simulink model "Commander_Stabilizer_QBot2e_Leader"  (Simulink 10.1)
settings: Solver=ode2  StartTime=0.0  StopTime=inf  FixedStep=0.002  RelTol=1e-3  EnableMultiTasking=on
model workspace (MAT data in the model file):
  Sig = Simulink.Signal
  Sig.DataType = 'auto'
  Sig.Dimensions = -1
  Sig.DimensionsMode = 'auto'
  Sig.Complexity = 'auto'
  Sig.SampleTime = -1
  Sig.SamplingMode = 'auto'
  video_step_size = 0.06
undefined symbols (not defined in the file): datetime, HIL, m, QBot2e_Commander_, QBot2e_Stabilizer_, saved_data
libraries: quarc_library x25, simulink x7
settings Model: Creator=Admin  LastModifiedBy=glai  SimulationMode=external
settings SolverCC: PositivePriorityOrder=on
settings DataIOCC: SaveFormat=Dataset
settings OptimizationCC: LifeSpan=auto
settings DebuggingCC: UnderspecifiedInitializationDetection=Simplified  MergeDetectMultiDrivingBlocksExec=error  ParameterPrecisionLossMsg=none
settings HardwareCC: ProdLargestAtomicInteger=Long  ProdLargestAtomicFloat=Double  ProdIntDivRoundTo=Zero  ProdEndianess=LittleEndian  ProdHWDeviceType=ARM Compatible->ARM Cortex
settings ModelReferenceCC: PropagateSignalLabelsOutOfModel=on
settings RTWCC: Description=QUARC Linux Raspberry Pi 3 Target (QBot 2e) Using Toolchain  SystemTargetFile=quarc_linux_pi_3.tlc  TemplateMakefile=quarc_default_tmf  Toolchain=QUARC linux_pi_3 | gmake (64-bit Windows)  BuildConfiguration=Faster Runs
settings STFCustomTargetCC: ConcurrentExecutionCompliant=on  UseToolchainInfoCompliant=on  SystemTargetFile=quarc_linux_pi_3.tlc
settings GRTTargetCC: ParMdlRefBuildCompliant=off  CompOptLevelCompliant=off  MatFileLogging=off  CPPClassGenCompliant=off  ExtMode=on  ExtModeMexFile=quarc_comm  ExtModeMexArgs='-w -d /tmp -uri %u -URI_Leader tcpip://localhost:18002 -URI_Host tcpip://192.168.2.H:18001','tcpip://192.168.2.Y:17001'
settings ConfigComp: CovHtmlReporting=off

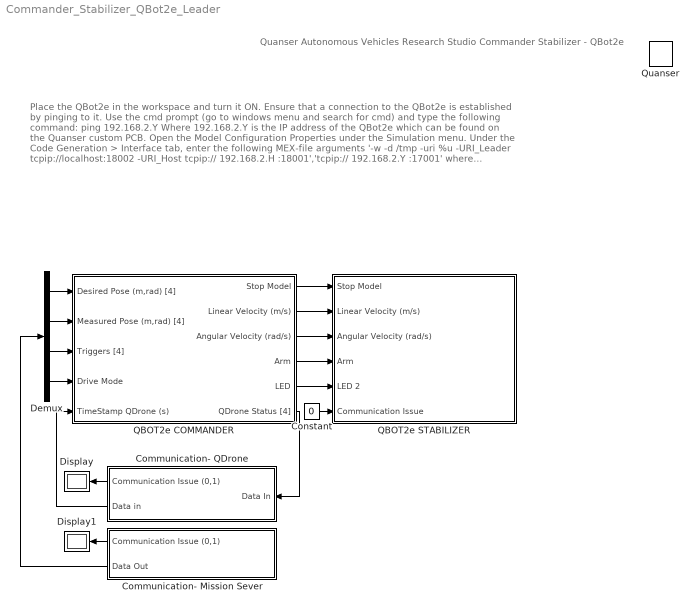
== system Commander_Stabilizer_QBot2e_Leader ==
  note: Quanser Autonomous Vehicles Research Studio
      | Commander Stabilizer - QBot2e
  note: Place the QBot2e in the workspace and turn it ON.
      | Ensure that a connection to the QBot2e is established by pinging to it. Use the cmd prompt (go to windows menu and search for cmd) and type the following command:
      | ping 192.168.2.Y
      | Where 192.168.2.Y is the IP address of the QBot2e which can be found on the Quanser custom PCB.
      |
      | Open the Model Configuration Properties under the Simulation menu.
      |
      | Under the Code Generation > Interface tab, enter the following MEX-file arguments
      | '-w -d /tmp -uri %u -URI_Leader tcpip://localhost:18002 -URI_Host tcpip:// 192.168.2.H :18001','tcpip:// 192.168.2.Y :17001'
      | where 192.168.2.H is the IP address of the ground control station PC (should be 192.168.2.5 by default), 192.168.2.Y is the IP address of the QBot2e which can be found on the custom Quanser PCB.
      |
      | Under the QUARC menu, click on Build .
      | NOTE : Ensure that the corresponding Mission_Server_Leader_Follower is running first before continuing.
      |
      | Under the QUARC menu, click on Start .
      |
      | You will hear a sequence of beeps, which indicate that the model has started running on the QBot 2e.
  "Communication- Mission Sever " : Subsystem
  Communication- QDrone : Subsystem
  Constant : Constant  Value=0
  Demux : Demux  Outputs=[ 4 4 4 1]
  Display : Display
  Display1 : Display
  QBOT2e COMMANDER : Subsystem
  QBOT2e STABILIZER : Subsystem
  Quanser : quarc_library/Logos/Quanser
  wires:
  QBOT2e COMMANDER/1(Stop Model) -> QBOT2e STABILIZER/1(Stop Model)
  QBOT2e COMMANDER/3(Angular Velocity (rad/s)) -> QBOT2e STABILIZER/3(Angular Velocity (rad/s))
  QBOT2e COMMANDER/4(Arm) -> QBOT2e STABILIZER/4(Arm)
  QBOT2e COMMANDER/2(Linear Velocity (m/s)) -> QBOT2e STABILIZER/2(Linear Velocity (m/s))
  QBOT2e COMMANDER/5(LED) -> QBOT2e STABILIZER/5(LED 2)
  "Communication- Mission Sever "/2(Data Out) -> Demux/1
  Demux/2 -> QBOT2e COMMANDER/2(Measured Pose (m,rad) [4])
  Demux/1 -> QBOT2e COMMANDER/1(Desired Pose (m,rad) [4])
  Constant/1 -> QBOT2e STABILIZER/6(Communication Issue)
  Demux/3 -> QBOT2e COMMANDER/3(Triggers [4])
  Demux/4 -> QBOT2e COMMANDER/4("Drive Mode ")
  QBOT2e COMMANDER/6(QDrone Status [4]) -> Communication- QDrone/1(Data In)
  Communication- QDrone/1(Communication Issue (0,1)) -> Display/1
  "Communication- Mission Sever "/1(Communication Issue (0,1)) -> Display1/1
  Communication- QDrone/2(Data in) -> QBOT2e COMMANDER/5(TimeStamp QDrone (s))

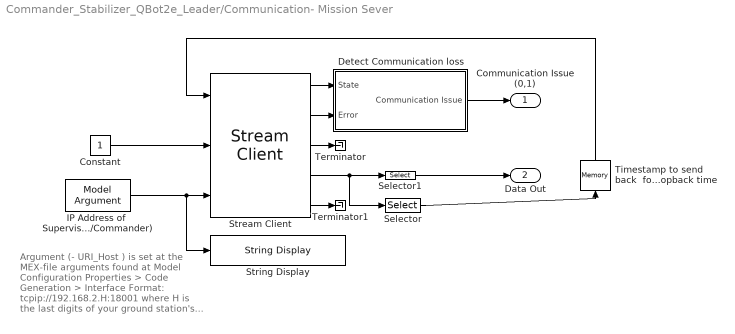
== system Commander_Stabilizer_QBot2e_Leader/Communication- Mission Sever  ==
  note: Argument (- URI_Host ) is set at the MEX-file arguments found at Model Configuration Properties > Code Generation > Interface
      |
      | Format:
      | tcpip://192.168.2.H:18001
      | where H is the last digits of your ground station's IP address (use ipconfig in a command prompt to find it out).
  Constant : Constant
  Detect Communication loss : Subsystem
  IP Address of  Supervisory Model (Mission Operator/Commander) : quarc_library/Sources/Signals/Model Argument  argument_name=URI_Host  has_value=on  data_type_mode=Specify via dialog  data_type=char  max_length=80  default_value=0  default_string=tcpip://192.168.2.H:18001  variable_size=off
      settings: AttributesFormatString=(-%<argument_name>)  SourceProductName=QUARC Targets
  Selector : Selector  InputPortWidth=14  IndexOptions=Index vector (dialog)  Indices=[14]  OutputSizes=1
  Selector1 : Selector  InputPortWidth=14  IndexOptions=Index vector (dialog)  Indices=[1:13]  OutputSizes=1
  Stream Client : quarc_library/Communications/Basic/Stream Client  uri_source=External input port  uri=tcpip://localhost:18999  apply_uri_to_all_configs=on  send_buffer_size=1460  receive_buffer_size=1460  byte_order=little endian (Intel - LSB first)  optimization=Minimum latency  send_options=Send most recent data  receive_options=Receive most recent data  default_value=zeros(1,14)  sample_time=qc_get_step_size  active=off  implementation=Use blocking I/O in a separate thread  send_fifo_size=1  receive_fifo_size=1  send_priority=0  receive_priority=0  send_dimensions=off  receive_dimensions=off  max_dimensions=-1  data_type=double  type_expr=BusObject
      settings: SourceProductName=The database C:\Users\user\AppData\Roaming\MathWorks\MATLAB\R2017a\slblocks_master.db is locked, or a table in the database is locked. (database is locked)
  String Display : quarc_library/Strings/String Display  alignment=center  display_mode=Single line  sample_time=-1  use_new=off
      settings: SourceProductName=QUARC Targets
  Terminator : Terminator
  Terminator1 : Terminator
  "Timestamp to send back  for loopback time " : Memory
  Communication Issue (0,1) : Outport  VectorParamsAs1DForOutWhenUnconnected=off
  Data Out : Outport  Port=2  VectorParamsAs1DForOutWhenUnconnected=off
  wires:
  Stream Client/5 -> Terminator1/1
  Constant/1 -> Stream Client/2
  Stream Client/3 -> Terminator/1
  IP Address of  Supervisory Model (Mission Operator/Commander)/1 -> String Display/1, Stream Client/3
  Stream Client/1 -> Detect Communication loss/1(State)
  Stream Client/2 -> Detect Communication loss/2(Error)
  Detect Communication loss/1(Communication Issue) -> Communication Issue (0,1)/1
  "Timestamp to send back  for loopback time "/1 -> Stream Client/1
  Selector/1 -> "Timestamp to send back  for loopback time "/1
  Stream Client/4 -> Selector1/1, Selector/1
  Selector1/1 -> Data Out/1

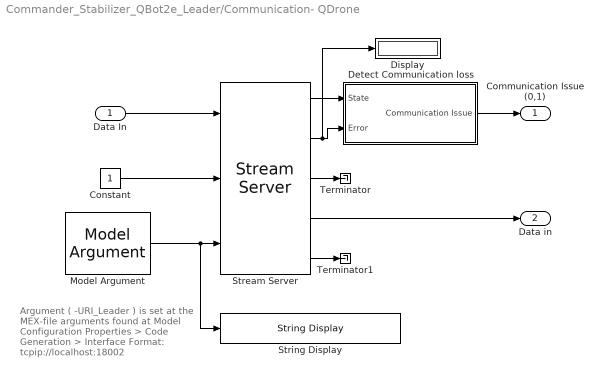
== system Commander_Stabilizer_QBot2e_Leader/Communication- QDrone ==
  note: Argument ( -URI_Leader ) is set at the MEX-file arguments
      | found at Model Configuration Properties > Code Generation > Interface
      |
      | Format:
      | tcpip://localhost:18002
  Data In : Inport
  Constant : Constant
  Detect Communication loss : Subsystem
  Display : Display
  Model Argument : quarc_library/Sources/Signals/Model Argument  argument_name=URI_Leader  has_value=on  data_type_mode=Specify via dialog  data_type=char  max_length=80  default_value=0  default_string=tcpip://localhost:18002  variable_size=off
      settings: AttributesFormatString=(-%<argument_name>)  SourceProductName=QUARC Targets
  Stream Server : quarc_library/Communications/Basic/Stream Server  uri_source=External input port  uri=tcpip://localhost:18001  apply_uri_to_all_configs=on  send_buffer_size=1460  receive_buffer_size=1460  byte_order=little endian (Intel - LSB first)  optimization=Minimum latency  send_options=Send most recent data  receive_options=Receive most recent data  default_value=zeros(1,1)  sample_time=qc_get_step_size  active=off  implementation=Use blocking I/O in a separate thread  send_fifo_size=1000  receive_fifo_size=1000  send_priority=0  receive_priority=0  send_dimensions=off  receive_dimensions=off  max_dimensions=-1  data_type=Inherited via back propagation  type_expr=BusObject
  "String Display " : quarc_library/Strings/String Display  alignment=center  display_mode=Single line  sample_time=-1  use_new=off
      settings: SourceProductName=QUARC Targets
  Terminator : Terminator
  Terminator1 : Terminator
  Communication Issue (0,1) : Outport  VectorParamsAs1DForOutWhenUnconnected=off
  Data in : Outport  Port=2  VectorParamsAs1DForOutWhenUnconnected=off
  wires:
  Detect Communication loss/1(Communication Issue) -> Communication Issue (0,1)/1
  Data In/1 -> Stream Server/1
  Stream Server/2 -> Display/1, Detect Communication loss/2(Error)
  Stream Server/1 -> Detect Communication loss/1(State)
  Stream Server/3 -> Terminator/1
  Constant/1 -> Stream Server/2
  Stream Server/5 -> Terminator1/1
  Stream Server/4 -> Data in/1
  Model Argument/1 -> Stream Server/3, "String Display "/1

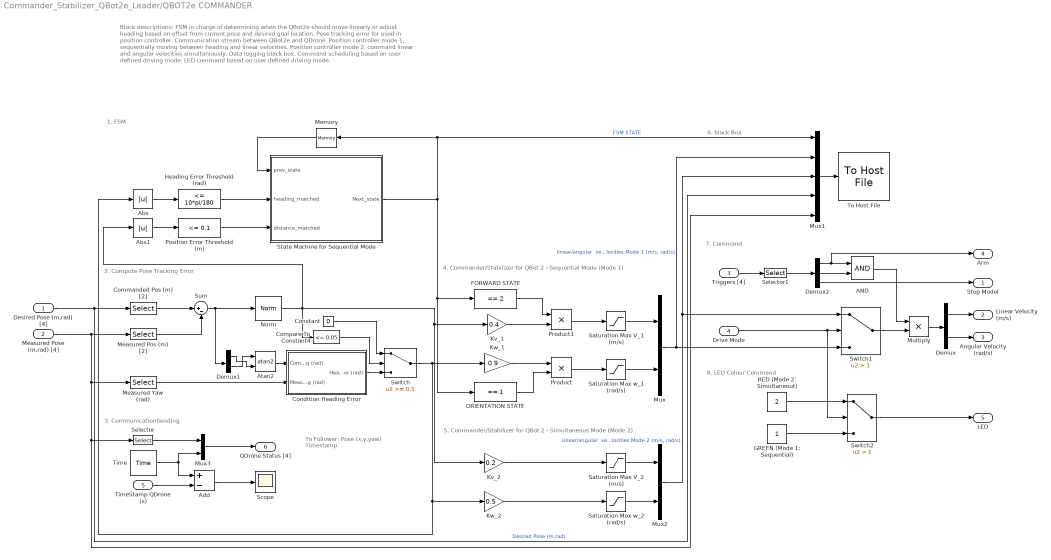
== system Commander_Stabilizer_QBot2e_Leader/QBOT2e COMMANDER ==
  note: Block descriptions:
      | FSM in charge of determining when the QBot2e should move linearly or adjust heading based on offset from current pose and desired goal location.
      | Pose tracking error for used in position controller.
      | Communication stream between QBot2e and QDrone.
      | Position controller mode 1, sequentially moving between heading and linear velocities.
      | Position controller mode 2, command linear and angular velocities simultaniously.
      | Data logging black box.
      | Command scheduling based on user defined driving mode.
      | LED command based on user defined driving mode.
  note: 7. Command
  note: To Follower:
      | Pose (x,y,yaw)
      | Timestamp
  note: 3. CommunicationSending
  note: 8. LED Colour Command
  note: 6. black Box
  note: 1. FSM
  note: 2. Compute Pose Tracking Error
  note: 5. Commander/Stabilizer for QBot 2 - Simultaneous Mode (Mode 2)
  note: 4. Commander/Stabilizer for QBot 2 - Sequential Mode (Mode 1)
  Desired Pose (m,rad) [4] : Inport
  Measured Pose (m,rad) [4] : Inport  Port=2
  Triggers [4] : Inport  Port=3
  "Drive Mode " : Inport  Port=4
  TimeStamp QDrone (s) : Inport  Port=5
  AND : Logic  AllPortsSameDT=off  OutDataTypeStr=boolean
  Abs : Abs
  Abs1 : Abs
  Add : Sum  Inputs=+-
  Atan2 : Trigonometry  Operator=atan2
  Commanded Pos (m) [2] : Selector  InputPortWidth=4  IndexOptions=Index vector (dialog)  Indices=[1,2]  OutputSizes=1
  Compare To Constant4 : simulink/Logic and Bit Operations/Compare To Constant  relop=<=  const=0.05  OutDataTypeStr=uint8
  Condition Heading Error : Subsystem
  Constant : Constant  Value=0
  Demux : Demux  Outputs=2
  Demux1 : Demux  Outputs=2
  Demux2 : Demux  Outputs=3
  FORWARD STATE : simulink/Logic and Bit Operations/Compare To Constant  relop===  const=2  OutDataTypeStr=uint8
  GREEN (Mode 1: Sequential) : Constant
  Heading Error Threshold (rad) : simulink/Logic and Bit Operations/Compare To Constant  relop=<=  const=10*pi/180  OutDataTypeStr=boolean
  Kv_1 : Gain  Gain=0.4
  Kv_2 : Gain  Gain=0.2
  Kw_1 : Gain  Gain=0.9
  Kw_2 : Gain  Gain=0.5
  Measured Pos (m) [2] : Selector  InputPortWidth=4  IndexOptions=Index vector (dialog)  Indices=[1,2]  OutputSizes=1
  Measured Yaw (rad) : Selector  InputPortWidth=4  IndexOptions=Index vector (dialog)  Indices=[4]  OutputSizes=1
  Memory : quarc_library/Discrete/Memory  initial_condition=0  sample_time=-1
      settings: SourceProductName=QUARC Targets
  Multiply : Product
  Mux : Mux  Inputs=2
  Mux1 : Mux  Inputs=5
  Mux2 : Mux  Inputs=2
  Mux3 : Mux  Inputs=2
  Norm : quarc_library/Math Operations/Vectors/Norm
      settings: SourceProductName=QUARC Targets
  ORIENTATION STATE : simulink/Logic and Bit Operations/Compare To Constant  relop===  const=1  OutDataTypeStr=uint8
  Position Error Threshold (m) : simulink/Logic and Bit Operations/Compare To Constant  relop=<=  const=0.1  OutDataTypeStr=boolean
  Product : Product
  Product1 : Product
  RED (Mode 2: Simultaneout) : Constant  Value=2
  Saturation Max V_1 (m/s) : Saturate
  Saturation Max V_2 (m/s) : Saturate
  Saturation Max w_1 (rad/s) : Saturate  UpperLimit=3  LowerLimit=-3
  Saturation Max w_2 (rad/s) : Saturate  UpperLimit=1  LowerLimit=-1
  Scope : Scope
  Selector : Selector  InputPortWidth=4  IndexOptions=Index vector (dialog)  Indices=[1,2,4]  OutputSizes=1
  Selector1 : Selector  InputPortWidth=4  IndexOptions=Index vector (dialog)  Indices=[1:3]  OutputSizes=1
  State Machine for Sequential Mode : MATLAB Function  TreatAsAtomicUnit=on
  Sum : Sum  Inputs=|+-
  Switch : Switch  Threshold=0.5
  Switch1 : Switch  Criteria=u2 > Threshold  Threshold=1
  Switch2 : Switch  Criteria=u2 > Threshold  Threshold=1
  Time : quarc_library/Sources/Time/Time  time_source=Wall clock  sample_time=qc_get_step_size
  To Host File : quarc_library/Sinks/To Host/To Host File  file_name=saved_data/%m/QBot2e_Commander_%{char(datetime)}.mat  variable_name=QBot2e_Commander  decimation=1  sample_time=-1  file_format=MAT-file v.5  options=No header or footer  append=off  final_file_name=saved_data/Commander_Stabilizer_QBot2e_Leader/QBot2e_Commander_2022-03-09 17-41-20.mat  bitrate=2000000
  Stop Model : Outport  VectorParamsAs1DForOutWhenUnconnected=off
  Linear Velocity (m/s) : Outport  Port=2  VectorParamsAs1DForOutWhenUnconnected=off
  Angular Velocity (rad/s) : Outport  Port=3  VectorParamsAs1DForOutWhenUnconnected=off
  Arm : Outport  Port=4  VectorParamsAs1DForOutWhenUnconnected=off
  LED : Outport  Port=5  VectorParamsAs1DForOutWhenUnconnected=off
  QDrone Status [4] : Outport  Port=6  VectorParamsAs1DForOutWhenUnconnected=off
  wires:
  Abs1/1 -> Position Error Threshold (m)/1
  Position Error Threshold (m)/1 -> State Machine for Sequential Mode/3(distance_matched)
  Memory/1 -> State Machine for Sequential Mode/1(prev_state)
  Heading Error Threshold (rad)/1 -> State Machine for Sequential Mode/2(heading_matched)
  Abs/1 -> Heading Error Threshold (rad)/1
  Demux1/2 -> Atan2/1
  Demux1/1 -> Atan2/2
  Compare To Constant4/1 -> Switch/2
  Atan2/1 -> Condition Heading Error/1(Commanded Heading (rad))
  Condition Heading Error/1(Heading Error (rad)) -> Switch/3
  Measured Yaw (rad)/1 -> Condition Heading Error/2(Measured Heading (rad))
  Desired Pose (m,rad) [4]/1 -> Mux1/4, Commanded Pos (m) [2]/1  "Desired Pose (m,rad)"
  Measured Pose (m,rad) [4]/1 -> Measured Pos (m) [2]/1, Mux1/5, Selector/1, Measured Yaw (rad)/1
  Constant/1 -> Switch/1
  Commanded Pos (m) [2]/1 -> Sum/1
  Measured Pos (m) [2]/1 -> Sum/2
  Sum/1 -> Norm/1, Demux1/1
  State Machine for Sequential Mode/1(Next_state) -> Memory/1, Mux1/1, ORIENTATION STATE/1, FORWARD STATE/1  "FSM STATE"
  Kv_1/1 -> Product1/2
  Product/1 -> Saturation Max w_1 (rad/s)/1
  Kw_1/1 -> Product/1
  FORWARD STATE/1 -> Product1/1
  ORIENTATION STATE/1 -> Product/2
  Product1/1 -> Saturation Max V_1 (m/s)/1
  Saturation Max w_1 (rad/s)/1 -> Mux/2
  Saturation Max V_1 (m/s)/1 -> Mux/1
  Demux/2 -> Angular Velocity (rad/s)/1
  Demux/1 -> Linear Velocity (m/s)/1
  Mux/1 -> Switch1/3, Mux1/2  "linear/angular  velocities Mode 1 (m/s, rad/s)"
  Switch/1 -> Abs/1, Kw_2/1, Kw_1/1
  Saturation Max V_2 (m/s)/1 -> Mux2/1
  Saturation Max w_2 (rad/s)/1 -> Mux2/2
  Kv_2/1 -> Saturation Max V_2 (m/s)/1
  Kw_2/1 -> Saturation Max w_2 (rad/s)/1
  Norm/1 -> Abs1/1, Kv_2/1, Kv_1/1, Compare To Constant4/1
  Mux2/1 -> Switch1/1, Mux1/3  "Linear/angular  velocities Mode 2 (m/s, rad/s)"
  Mux1/1 -> To Host File/1
  Multiply/1 -> Demux/1
  "Drive Mode "/1 -> Switch2/2, Switch1/2
  Switch2/1 -> LED/1
  RED (Mode 2: Simultaneout)/1 -> Switch2/1
  GREEN (Mode 1: Sequential)/1 -> Switch2/3
  Triggers [4]/1 -> Selector1/1
  Switch1/1 -> Multiply/2
  Demux2/2 -> AND/2
  Time/1 -> Add/1, Mux3/2
  Selector/1 -> Mux3/1
  Mux3/1 -> QDrone Status [4]/1
  Demux2/1 -> AND/1, Arm/1
  AND/1 -> Multiply/1
  Demux2/3 -> Stop Model/1
  TimeStamp QDrone (s)/1 -> Add/2
  Add/1 -> Scope/1
  Selector1/1 -> Demux2/1

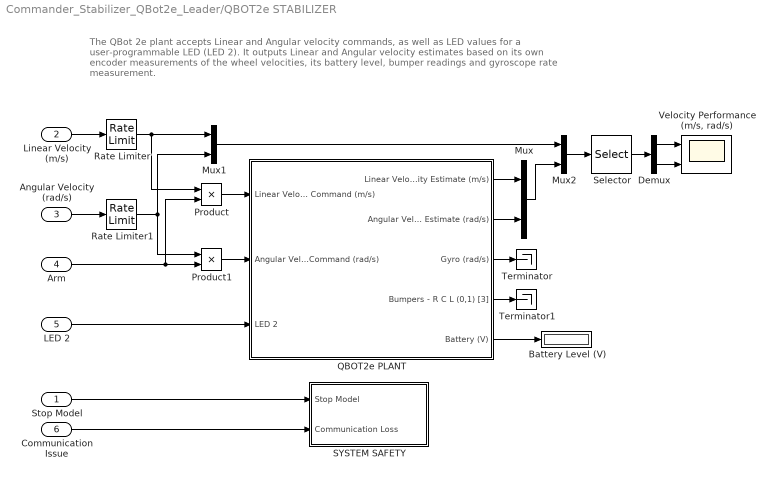
== system Commander_Stabilizer_QBot2e_Leader/QBOT2e STABILIZER ==
  note: The QBot 2e plant accepts Linear and Angular velocity commands, as well as LED values for a user-programmable LED (LED 2).
      | It outputs Linear and Angular velocity estimates based on its own encoder measurements of the wheel velocities, its battery level,
      | bumper readings and gyroscope rate measurement.
  Stop Model : Inport
  Linear Velocity (m/s) : Inport  Port=2
  Angular Velocity (rad/s) : Inport  Port=3
  Arm : Inport  Port=4
  LED 2 : Inport  Port=5
  Communication Issue : Inport  Port=6
  Battery Level (V) : Display
  Demux : Demux  Outputs=[2 2]
  Mux : Mux  Inputs=2
  Mux1 : Mux  Inputs=2
  Mux2 : Mux  Inputs=2
  Product : Product
  Product1 : Product
  QBOT2e PLANT : Subsystem
  Rate Limiter : RateLimiter  RisingSlewLimit=0.5  FallingSlewLimit=-0.5  SampleTimeMode=inherited
  Rate Limiter1 : RateLimiter  RisingSlewLimit=3  FallingSlewLimit=-3  SampleTimeMode=inherited
  SYSTEM SAFETY : Subsystem
  Selector : Selector  InputPortWidth=4  IndexOptions=Index vector (dialog)  Indices=[1 3 2 4]  OutputSizes=1
  Terminator : Terminator
  Terminator1 : Terminator
  "Velocity Performance (m/s, rad/s)" : Scope  NumInputPorts=2
  wires:
  Angular Velocity (rad/s)/1 -> Rate Limiter1/1
  Linear Velocity (m/s)/1 -> Rate Limiter/1
  Mux1/1 -> Mux2/1
  Mux2/1 -> Selector/1
  Selector/1 -> Demux/1
  Demux/1 -> "Velocity Performance (m/s, rad/s)"/1
  Demux/2 -> "Velocity Performance (m/s, rad/s)"/2
  Arm/1 -> Product1/2, Product/2
  Stop Model/1 -> SYSTEM SAFETY/1(Stop Model)
  Communication Issue/1 -> SYSTEM SAFETY/2(Communication Loss)
  Product1/1 -> QBOT2e PLANT/2(Angular Velocity Command (rad/s))
  Product/1 -> QBOT2e PLANT/1(Linear Velocity Command (m/s))
  LED 2/1 -> QBOT2e PLANT/3(LED 2)
  QBOT2e PLANT/5(Battery (V)) -> Battery Level (V)/1
  QBOT2e PLANT/2(Angular Velocity Estimate (rad/s)) -> Mux/2
  QBOT2e PLANT/1(Linear Velocity Estimate (m/s)) -> Mux/1
  Mux/1 -> Mux2/2
  QBOT2e PLANT/3(Gyro (rad/s)) -> Terminator/1
  QBOT2e PLANT/4(Bumpers - R C L (0,1) [3]) -> Terminator1/1
  Rate Limiter/1 -> Product/1, Mux1/1
  Rate Limiter1/1 -> Product1/1, Mux1/2

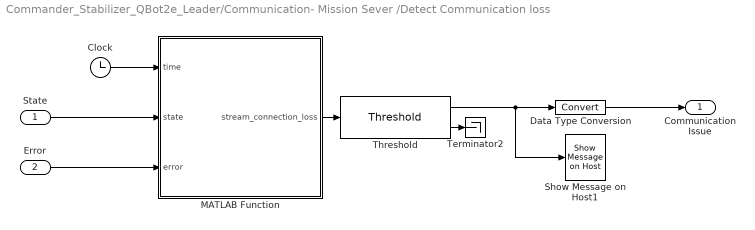
== system Commander_Stabilizer_QBot2e_Leader/Communication- Mission Sever /Detect Communication loss ==
  State : Inport
  Error : Inport  Port=2
  Clock : Clock
  Data Type Conversion : DataTypeConversion
  MATLAB Function : MATLAB Function  TreatAsAtomicUnit=on
  Show Message on Host1 : quarc_library/Sinks/Error Handling/Show Message on Host  message_type=Fixed error message  message_icon=Warning  message=Not connection between QBot2e and Mission Server
      settings: AttributesFormatString="\"%<message>\""  SourceProductName=QUARC Targets
  Terminator2 : Terminator
  Threshold : quarc_library/Discontinuities/Threshold  operator=>=  param_src=Specify via dialog  threshold=0.5  duration=0.1
      settings: SourceProductName=QUARC Targets
  Communication Issue : Outport  VectorParamsAs1DForOutWhenUnconnected=off
  wires:
  Error/1 -> MATLAB Function/3(error)
  MATLAB Function/1(stream_connection_loss) -> Threshold/1
  State/1 -> MATLAB Function/2(state)
  Clock/1 -> MATLAB Function/1(time)
  Threshold/1 -> Show Message on Host1/1, Data Type Conversion/1
  Threshold/2 -> Terminator2/1
  Data Type Conversion/1 -> Communication Issue/1

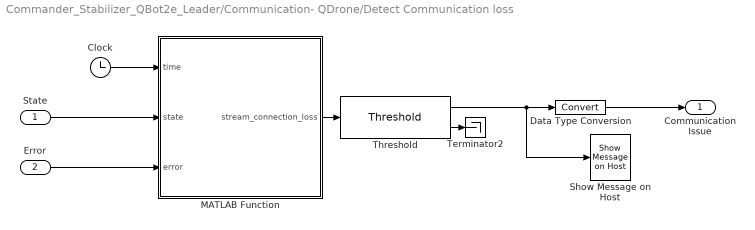
== system Commander_Stabilizer_QBot2e_Leader/Communication- QDrone/Detect Communication loss ==
  State : Inport
  Error : Inport  Port=2
  Clock : Clock
  Data Type Conversion : DataTypeConversion
  MATLAB Function : MATLAB Function  TreatAsAtomicUnit=on
  Show Message on Host : quarc_library/Sinks/Error Handling/Show Message on Host  message_type=Fixed error message  message_icon=Warning  message=No connection between QBot2e and QDrone
      settings: AttributesFormatString="\"%<message>\""  SourceProductName=QUARC Targets
  Terminator2 : Terminator
  Threshold : quarc_library/Discontinuities/Threshold  operator=>=  param_src=Specify via dialog  threshold=0.5  duration=0.1
      settings: SourceProductName=QUARC Targets
  Communication Issue : Outport  VectorParamsAs1DForOutWhenUnconnected=off
  wires:
  Data Type Conversion/1 -> Communication Issue/1
  Threshold/2 -> Terminator2/1
  Clock/1 -> MATLAB Function/1(time)
  State/1 -> MATLAB Function/2(state)
  MATLAB Function/1(stream_connection_loss) -> Threshold/1
  Error/1 -> MATLAB Function/3(error)
  Threshold/1 -> Show Message on Host/1, Data Type Conversion/1

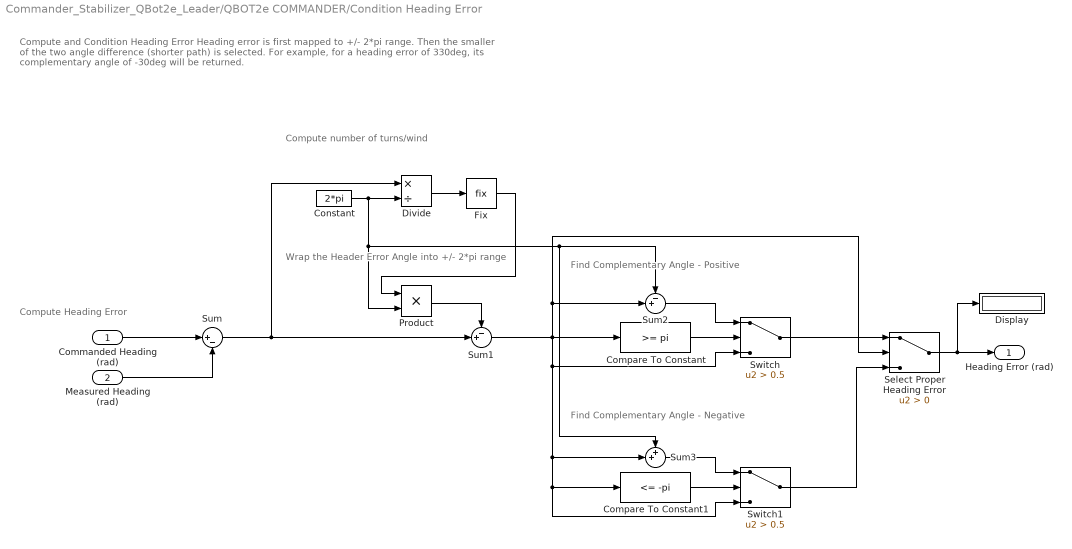
== system Commander_Stabilizer_QBot2e_Leader/QBOT2e COMMANDER/Condition Heading Error ==
  note: Find Complementary Angle - Negative
  note: Find Complementary Angle - Positive
  note: Wrap the Header Error Angle into +/- 2*pi range
  note: Compute number of turns/wind
  note: Compute Heading Error
  note: Compute and Condition Heading Error
      |
      | Heading error is first mapped to +/- 2*pi range.
      | Then the smaller of the two angle difference (shorter path) is selected.
      |
      | For example, for a heading error of 330deg, its complementary angle of -30deg will be returned.
  Commanded Heading (rad) : Inport
  Measured Heading (rad) : Inport  Port=2
  Compare To Constant : simulink/Logic and Bit Operations/Compare To Constant  relop=>=  const=pi  OutDataTypeStr=boolean
  Compare To Constant1 : simulink/Logic and Bit Operations/Compare To Constant  relop=<=  const=-pi  OutDataTypeStr=boolean
  Constant : Constant  Value=2*pi
  Display : Display
  Divide : Product  Inputs=*/
  Fix : Rounding  Operator=fix
  Product : Product
  Select Proper Heading Error : Switch  Criteria=u2 > Threshold
  Sum : Sum  Inputs=|+-
  Sum1 : Sum  Inputs=-+|
  Sum2 : Sum  Inputs=-+|
  Sum3 : Sum  Inputs=++|
  Switch : Switch  Criteria=u2 > Threshold  Threshold=0.5
  Switch1 : Switch  Criteria=u2 > Threshold  Threshold=0.5
  Heading Error (rad) : Outport  VectorParamsAs1DForOutWhenUnconnected=off
  wires:
  Commanded Heading (rad)/1 -> Sum/1
  Measured Heading (rad)/1 -> Sum/2
  Divide/1 -> Fix/1
  Sum/1 -> Sum1/2, Divide/1
  Product/1 -> Sum1/1
  Fix/1 -> Product/1
  Compare To Constant/1 -> Switch/2
  Sum1/1 -> Sum2/2, Select Proper Heading Error/2, Sum3/2, Compare To Constant1/1, Switch1/3, Switch/3, Compare To Constant/1
  Sum2/1 -> Switch/1
  Constant/1 -> Sum3/1, Sum2/1, Product/2, Divide/2
  Compare To Constant1/1 -> Switch1/2
  Sum3/1 -> Switch1/1
  Switch/1 -> Select Proper Heading Error/1
  Switch1/1 -> Select Proper Heading Error/3
  Select Proper Heading Error/1 -> Heading Error (rad)/1, Display/1

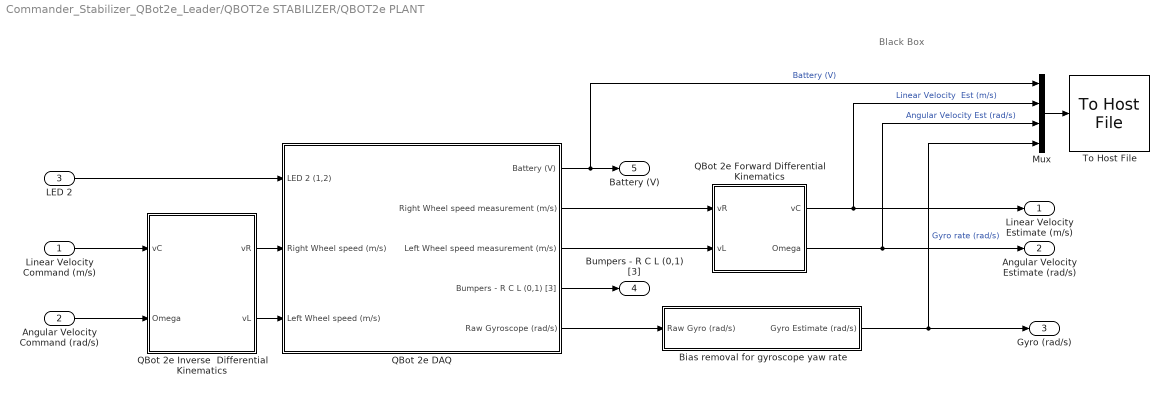
== system Commander_Stabilizer_QBot2e_Leader/QBOT2e STABILIZER/QBOT2e PLANT ==
  note: Black Box
  Linear Velocity Command (m/s) : Inport
  Angular Velocity Command (rad/s) : Inport  Port=2
  LED 2 : Inport  Port=3
  Bias removal for gyroscope yaw rate : Subsystem
  Mux : Mux
  QBot 2e DAQ : Subsystem
  QBot 2e Forward Differential Kinematics : MATLAB Function  TreatAsAtomicUnit=on
  QBot 2e Inverse  Differential Kinematics : MATLAB Function  TreatAsAtomicUnit=on
  To Host File : quarc_library/Sinks/To Host/To Host File  file_name=saved_data/%m/QBot2e_Stabilizer_%{char(datetime)}.mat  variable_name=QBot2e_Stabilizer  decimation=1  sample_time=-1  file_format=MAT-file v.5  options=No header or footer  append=off  final_file_name=saved_data/Commander_Stabilizer_QBot2e_Leader/QBot2e_Stabilizer_2022-03-09 17-41-30.mat  bitrate=2000000
  Linear Velocity Estimate (m/s) : Outport  VectorParamsAs1DForOutWhenUnconnected=off
  Angular Velocity Estimate (rad/s) : Outport  Port=2  VectorParamsAs1DForOutWhenUnconnected=off
  Gyro (rad/s) : Outport  Port=3  VectorParamsAs1DForOutWhenUnconnected=off
  Bumpers - R C L (0,1) [3] : Outport  Port=4  VectorParamsAs1DForOutWhenUnconnected=off
  Battery (V) : Outport  Port=5  VectorParamsAs1DForOutWhenUnconnected=off
  wires:
  Angular Velocity Command (rad/s)/1 -> QBot 2e Inverse  Differential Kinematics/2(Omega)
  Linear Velocity Command (m/s)/1 -> QBot 2e Inverse  Differential Kinematics/1(vC)
  QBot 2e Forward Differential Kinematics/1(vC) -> Mux/2, Linear Velocity Estimate (m/s)/1  "Linear Velocity  Est (m/s)"
  QBot 2e Forward Differential Kinematics/2(Omega) -> Mux/3, Angular Velocity Estimate (rad/s)/1  "Angular Velocity Est (rad/s)"
  Bias removal for gyroscope yaw rate/1(Gyro Estimate (rad/s)) -> Mux/4, Gyro (rad/s)/1  "Gyro rate (rad/s)"
  LED 2/1 -> QBot 2e DAQ/1(LED 2 (1,2))
  QBot 2e DAQ/1(Battery (V)) -> Battery (V)/1, Mux/1  "Battery (V)"
  QBot 2e DAQ/2(Right Wheel speed measurement (m/s)) -> QBot 2e Forward Differential Kinematics/1(vR)
  QBot 2e DAQ/3(Left Wheel speed measurement (m/s)) -> QBot 2e Forward Differential Kinematics/2(vL)
  QBot 2e DAQ/4(Bumpers - R C L (0,1) [3]) -> Bumpers - R C L (0,1) [3]/1
  QBot 2e DAQ/5(Raw Gyroscope (rad/s)) -> Bias removal for gyroscope yaw rate/1(Raw Gyro (rad/s))
  QBot 2e Inverse  Differential Kinematics/1(vR) -> QBot 2e DAQ/2(Right Wheel speed (m/s))
  QBot 2e Inverse  Differential Kinematics/2(vL) -> QBot 2e DAQ/3(Left Wheel speed (m/s))
  Mux/1 -> To Host File/1

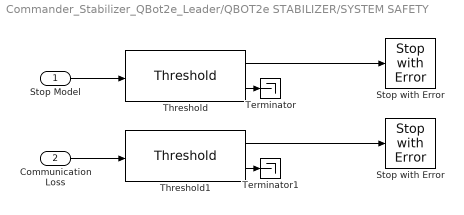
== system Commander_Stabilizer_QBot2e_Leader/QBOT2e STABILIZER/SYSTEM SAFETY ==
  Stop Model : Inport
  Communication Loss : Inport  Port=2
  Stop with Error : quarc_library/Sinks/Error Handling/Stop with Error  message_type=Fixed error message  message=QBot 2e Stabilizer: Operator Stopped Model
      settings: AttributesFormatString="\"%<message>\""  SourceProductName=QUARC Targets
  "Stop with Error " : quarc_library/Sinks/Error Handling/Stop with Error  message_type=Fixed error message  message=QBot 2e Stabilizer: Communication Issue with Operator
      settings: AttributesFormatString="\"%<message>\""  SourceProductName=QUARC Targets
  Terminator : Terminator
  Terminator1 : Terminator
  Threshold : quarc_library/Discontinuities/Threshold  operator=>  param_src=Specify via dialog  threshold=0.5  duration=2
      settings: SourceProductName=QUARC Targets
  Threshold1 : quarc_library/Discontinuities/Threshold  operator=>  param_src=Specify via dialog  threshold=0.5  duration=3
      settings: SourceProductName=QUARC Targets
  wires:
  Threshold/1 -> Stop with Error/1
  Communication Loss/1 -> Threshold1/1
  Threshold1/1 -> "Stop with Error "/1
  Threshold1/2 -> Terminator1/1
  Stop Model/1 -> Threshold/1
  Threshold/2 -> Terminator/1

== system Commander_Stabilizer_QBot2e_Leader/QBOT2e STABILIZER/QBOT2e PLANT/Bias removal for gyroscope yaw rate ==
  Raw Gyro (rad/s) : Inport
  Bias Removal : quarc_library/Discrete/Bias Removal  start_time=3  end_time=4  switch_id=0  sample_time=qc_get_step_size
      settings: SourceProductName=QUARC Targets
  Product : Product  RndMeth=Zero
  Terminator7 : Terminator
  Gyro Estimate (rad/s) : Outport  VectorParamsAs1DForOutWhenUnconnected=off
  wires:
  Bias Removal/3 -> Product/2
  Bias Removal/2 -> Terminator7/1
  Raw Gyro (rad/s)/1 -> Bias Removal/1
  Product/1 -> Gyro Estimate (rad/s)/1
  Bias Removal/1 -> Product/1

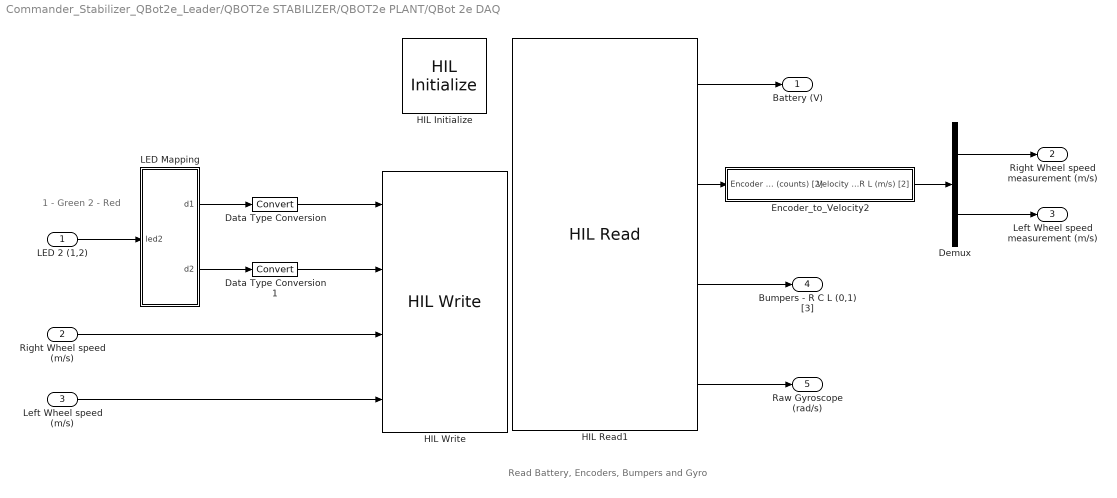
== system Commander_Stabilizer_QBot2e_Leader/QBOT2e STABILIZER/QBOT2e PLANT/QBot 2e DAQ ==
  note: 1 - Green
      | 2 - Red
  note: Read Battery, Encoders, Bumpers and Gyro
  LED 2 (1,2) : Inport
  Right Wheel speed (m/s) : Inport  Port=2
  Left Wheel speed (m/s) : Inport  Port=3
  Data Type Conversion : DataTypeConversion
  Data Type Conversion1 : DataTypeConversion
  Demux : Demux  Outputs=2
  Encoder_to_Velocity2 : Subsystem
  HIL Initialize : quarc_library/Data Acquisition/Generic/Configuration/HIL Initialize  Priority=-99  object_name=HIL-1  board_type=qbot2e  board_number=0  board_options=pwm0_en=1;pwm0_pin=12;pwm1_en=1;pwm1_pin=13;  exclusive=off  active=off  hardware_clocks=[]  clock_modes=[]  initial_clock_frequencies=[]  set_clock_params_at_start=off  set_clock_params_at_switch_in=off  set_clock_frequencies_at_start=off  set_clock_frequencies_at_switch_in=off  analog_input_channels=[0:5]  analog_input_configurations=[]  analog_input_maximums=[16.5 3.3 3.3 3.3 3.3 3.3]  analog_input_minimums=[0 0 0 0 0 0]  set_analog_input_params_at_start=off  set_analog_input_params_at_switch_in=off  analog_output_channels=[]  analog_output_maximums=[]  analog_output_minimums=[]  initial_analog_outputs=[]  final_analog_outputs=[]  watchdog_analog_outputs=[]  set_analog_output_params_at_start=off  set_analog_output_params_at_switch_in=off  set_analog_outputs_at_start=off  set_analog_outputs_at_switch_in=off  set_analog_outputs_at_terminate=off  set_analog_outputs_at_switch_out=off  set_analog_outputs_on_watchdog=off  digital_input_channels=[28:58]  digital_output_channels=[28:31]  digital_output_configuration=[]  initial_digital_outputs=[0]  final_digital_outputs=[0]  watchdog_digital_outputs=[]  set_digital_output_params_at_start=off  set_digital_output_params_at_switch_in=off  set_digital_outputs_at_start=on  set_digital_outputs_at_switch_in=off  set_digital_outputs_at_terminate=on  set_digital_outputs_at_switch_out=off  set_digital_outputs_on_watchdog=off  encoder_channels=[0:1]  quadrature=[4]  encoder_filter_frequency=[]  initial_encoder_counts=[0]  set_encoder_params_at_start=on  set_encoder_params_at_switch_in=off  set_encoder_counts_at_start=on  set_encoder_counts_at_switch_in=off  pwm_channels=[0:1]  pwm_modes=0  pwm_frequency=[20e6/1024]  pwm_configuration=[0]  pwm_alignment=[0]  pwm_polarity=[1]  pwm_leading_deadband=[]  pwm_trailing_deadband=[]  initial_pwm_outputs=[0]  final_pwm_outputs=[0]  watchdog_pwm_outputs=[]  set_pwm_params_at_start=on  set_pwm_params_at_switch_in=off  set_pwm_outputs_at_start=on  set_pwm_outputs_at_switch_in=off  set_pwm_outputs_at_terminate=on  set_pwm_outputs_at_switch_out=off  set_pwm_outputs_on_watchdog=off  other_output_channels=[2000:2001 14000 16000]  initial_other_outputs=[0 0 0 7]  final_other_outputs=[0 0 0 7]  watchdog_other_outputs=[]  set_other_outputs_at_start=on  set_other_outputs_at_switch_in=off  set_other_outputs_at_terminate=on  set_other_outputs_at_switch_out=off  set_other_outputs_on_watchdog=off
  HIL Read1 : quarc_library/Data Acquisition/Generic/Immediate I//O/HIL Read  object_name=HIL-1  analog_channels=[0]  encoder_channels=[0:1]  digital_channels=[28:30]  other_channels=[1002]  sample_time=qc_get_step_size  active=on  vector_output=on  data_type_mode=Inherit via back propagation  encoder_data_type=double  digital_data_type=boolean
  HIL Write : quarc_library/Data Acquisition/Generic/Immediate I//O/HIL Write  object_name=HIL-1  analog_channels=[]  pwm_channels=[]  digital_channels=[30:31]  other_channels=[2000:2001]  sample_time=qc_get_step_size  active=on  vector_input=off
  LED Mapping : MATLAB Function  TreatAsAtomicUnit=on
  Battery (V) : Outport  VectorParamsAs1DForOutWhenUnconnected=off
  Right Wheel speed measurement (m/s) : Outport  Port=2  VectorParamsAs1DForOutWhenUnconnected=off
  Left Wheel speed measurement (m/s) : Outport  Port=3  VectorParamsAs1DForOutWhenUnconnected=off
  Bumpers - R C L (0,1) [3] : Outport  Port=4  VectorParamsAs1DForOutWhenUnconnected=off
  Raw Gyroscope (rad/s) : Outport  Port=5  VectorParamsAs1DForOutWhenUnconnected=off
  wires:
  HIL Read1/3 -> Bumpers - R C L (0,1) [3]/1
  LED Mapping/1(d1) -> Data Type Conversion/1
  HIL Read1/2 -> Encoder_to_Velocity2/1(Encoder - R L (counts) [2])
  LED Mapping/2(d2) -> Data Type Conversion1/1
  Encoder_to_Velocity2/1(Velocity - R L (m/s) [2]) -> Demux/1
  LED 2 (1,2)/1 -> LED Mapping/1(led2)
  Demux/1 -> Right Wheel speed measurement (m/s)/1
  Demux/2 -> Left Wheel speed measurement (m/s)/1
  HIL Read1/1 -> Battery (V)/1
  HIL Read1/4 -> Raw Gyroscope (rad/s)/1
  Data Type Conversion/1 -> HIL Write/1
  Right Wheel speed (m/s)/1 -> HIL Write/3
  Left Wheel speed (m/s)/1 -> HIL Write/4
  Data Type Conversion1/1 -> HIL Write/2

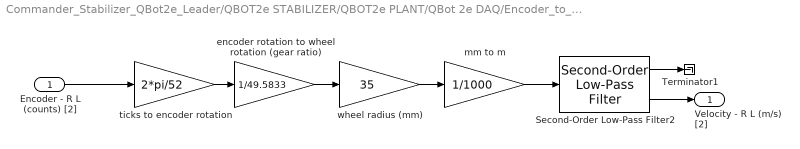
== system Commander_Stabilizer_QBot2e_Leader/QBOT2e STABILIZER/QBOT2e PLANT/QBot 2e DAQ/Encoder_to_Velocity2 ==
  Encoder - R L (counts) [2] : Inport
  " encoder rotation to wheel rotation (gear ratio)" : Gain  Gain=1/49.5833
  Second-Order Low-Pass Filter2 : quarc_library/Continuous/Second-Order Low-Pass Filter  params_source=Internal (dialog parameters)  input_width=10  input_zeta=1  input_init=0
  Terminator1 : Terminator
  mm to m : Gain  Gain=1/1000
  ticks to encoder rotation : Gain  Gain=2*pi/52
  wheel radius (mm) : Gain  Gain=35
  Velocity - R L (m/s) [2] : Outport  VectorParamsAs1DForOutWhenUnconnected=off
  wires:
  Second-Order Low-Pass Filter2/1 -> Terminator1/1
  mm to m/1 -> Second-Order Low-Pass Filter2/1
  Second-Order Low-Pass Filter2/2 -> Velocity - R L (m/s) [2]/1
  wheel radius (mm)/1 -> mm to m/1
  ticks to encoder rotation/1 -> " encoder rotation to wheel rotation (gear ratio)"/1
  Encoder - R L (counts) [2]/1 -> ticks to encoder rotation/1
  " encoder rotation to wheel rotation (gear ratio)"/1 -> wheel radius (mm)/1

== matlab function QBOT2e STABILIZER/QBOT2e PLANT/QBot 2e DAQ/LED Mapping ==
  data: d1 output double; led2 input double; d2 output double
function [d1, d2] = fcn(led2)


% Default LEDs are both OFF.
d1 = 0;
d2 = 0;

if led2 == 1
    d2 = 1;
elseif led2 == 2
    d1 = 1;
end

== matlab function QBOT2e STABILIZER/QBOT2e PLANT/QBot 2e Forward Differential Kinematics ==
  data: vR input double; vL input double; vC output double; Omega output double
function [vC,Omega] = qbot_i_d_k(vR,vL)

d= 0.235; % wheel base

vC = 0.5*(vL+vR); 
Omega = (1/d)*(vR-vL);

== matlab function Communication- Mission Sever /Detect Communication loss/MATLAB Function ==
  data: time input double; stream_connection_loss output double; state input double; error input double
function stream_connection_loss  = fcn(time, state, error)

stream_connection_loss = 0;
if time > 3
    if ((state ~= 2)&&(error < 0))
        % stream connection is not established correctly
        stream_connection_loss = 1;
    end
end

== matlab function QBOT2e COMMANDER/State Machine for Sequential Mode ==
  data: prev_state input double; Next_state output double; heading_matched input double; distance_matched input double
function Next_state  = fcn(prev_state,heading_matched, distance_matched)

Next_state = prev_state;
switch prev_state
    
    case 0 % IDLE/Stationary - QBot not moving
        if ~distance_matched
            if ~heading_matched
                Next_state = 1; % Adjust heading first
            else
                Next_state = 2; % Move towards target position
            end
        end
    case 1  % ORIENTATION TURNING
        if heading_matched
            if ~distance_matched
                Next_state = 2; % Move towards target position
            else
                Next_state = 0; % Done. Back to IDLE
            end
        end
    case 2  % MOVING TO TARGET
            if ~heading_matched
                Next_state = 1; % Adjust heading first
            elseif distance_matched
            %if distance_matched
                Next_state = 0; % Done. Back to IDLE
            end
end






end

== matlab function Communication- QDrone/Detect Communication loss/MATLAB Function ==
  data: time input double; stream_connection_loss output double; state input double; error input double
function stream_connection_loss  = fcn(time, state, error)

stream_connection_loss = 0;
if time > 3
    if ((state ~= 2)&&(error <= 0))
        % stream connection is not established correctly
        stream_connection_loss = 1;
    end
end

== matlab function QBOT2e STABILIZER/QBOT2e PLANT/QBot 2e Inverse Differential Kinematics ==
  data: vR output double; vL output double; vC input double; Omega input double
function [vR,vL] = qbot_f_d_k(vC , Omega)

d=0.235; % wheel base

vR = vC + Omega*d/2; % right wheel velocity
vL= vC - Omega*d/2; % left wheel velocity
